simulink model "Praktikum06"  (R2023b)
settings: Solver=VariableStepAuto  StartTime=0.0  StopTime=0.01  RelTol=1e-3
model workspace (MAT data in the model file):
  CodeRate = 0.75
  M = 16
  PunctureVector = [1; 1; 0; 1; 0; 1]
  TracebackDepth = 48
  Trelli.numInputSymbols = 2
  Trelli.numOutputSymbols = 4
  Trelli.numStates = 64
  Trelli.nextStates = [0  32; 0  32; 1  33; 1  33; 2  34; 2  34; 3  35; 3  35; 4  36; 4  36; 5  37; 5  37; 6  38; 6  38; 7  39; 7  39; 8  40; 8  40; 9  41; 9  41; 10  42; 10  42; 11  43; 11  43; 12  44; 12  44; 13  45; 13  45; 14  46; 14  46; 15  47; 15  47; 16  48; 16  48; 17  49; 17  49; 18  50; 18  50; 19  51; 19  51; 20  52; 20  52; 21  53; 21  53; 22  54; 22  54; 23  55; 23  55; 24  56; 24  56; 25  57; 25  57; 26  58; 26  58; 27  59; 27  59; 28  60; 28  60; 29  61; 29  61; 30  62; 30  62; 31  63; 31  63]
  Trelli.outputs = [0  3; 3  0; 1  2; 2  1; 0  3; 3  0; 1  2; 2  1; 3  0; 0  3; 2  1; 1  2; 3  0; 0  3; 2  1; 1  2; 3  0; 0  3; 2  1; 1  2; 3  0; 0  3; 2  1; 1  2; 0  3; 3  0; 1  2; 2  1; 0  3; 3  0; 1  2; 2  1; 2  1; 1  2; 3  0; 0  3; 2  1; 1  2; 3  0; 0  3; 1  2; 2  1; 0  3; 3  0; 1  2; 2  1; 0  3; 3  0; 1  2; 2  1; 0  3; 3  0; 1  2; 2  1; 0  3; 3  0; 2  1; 1  2; 3  0; 0  3; 2  1; 1  2; 3  0; 0  3]
  Ts = 5e-08
undefined symbols (not defined in the file): doppler, magnitude
libraries: dspxfrm3 x3, commchan3 x2, commrflib2 x2, commcnvcod2 x2, commdigbbndam3 x2, dspindex x2, dspsigops x2, commrandsrc3 x1, commsink2 x1, dspstat3 x1, dspmathops x1, dspquant2 x1
settings Model: Creator=suttarar@hu-berlin.de  LastModifiedBy=suttarar@hu-berlin.de

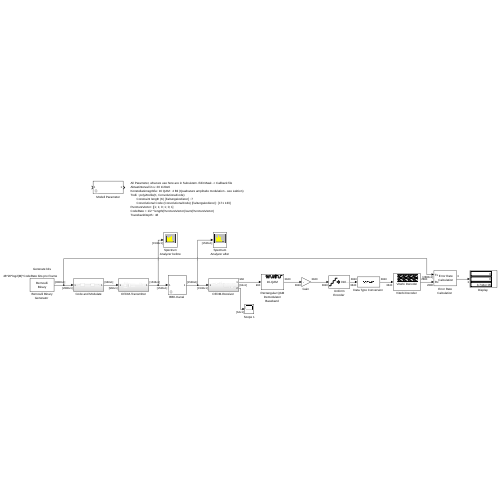
[thumbnail: Simulink's stored preview of the top-level diagram]
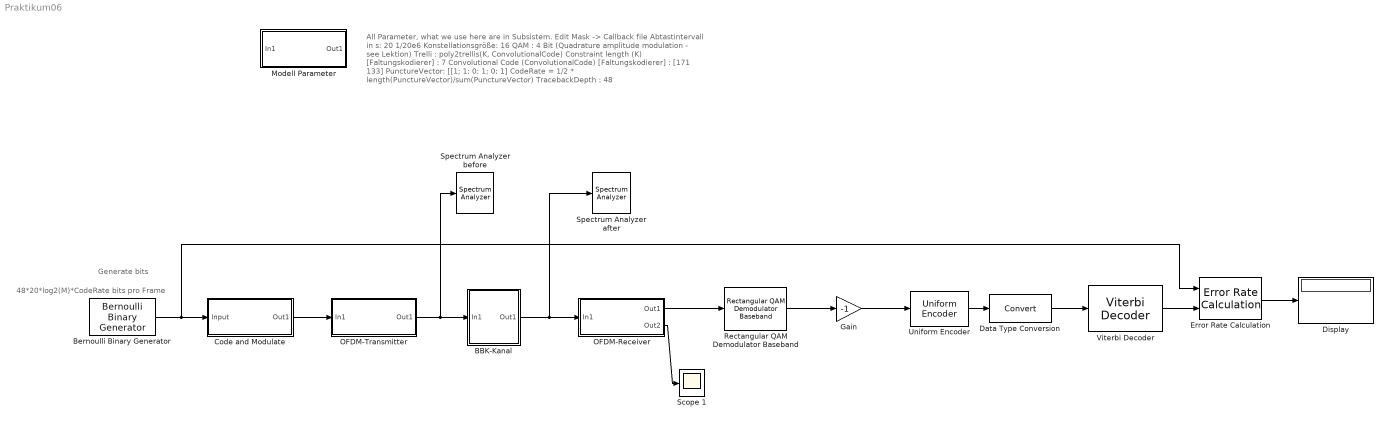
== system Praktikum06 ==
  note: All Parameter, what we use here are in Subsistem. Edit Mask -> Callback file
      | Abtastintervall in s: 20 1/20e6
      | Konstellationsgröße: 16 QAM : 4 Bit (Quadrature amplitude modulation - see Lektion)
      | Trelli : poly2trellis(K, ConvolutionalCode)
      | Constraint length (K) [Faltungskodierer] : 7
      | Convolutional Code (ConvolutionalCode) [Faltungskodierer] : [171 133]
      | PunctureVector: [[1; 1; 0; 1; 0; 1]
      | CodeRate = 1/2 * length(PunctureVector)/sum(PunctureVector)
      | TracebackDepth : 48
  note: 48*20*log2(M)*CodeRate bits pro Frame
  note: Generate bits
  "BBK-Kanal " : Subsystem  mask{MaxDoppler=0, PathDelays=0, PathGains=0, EnableMultipath=0, PathLoss=0, FrequencyOffset=0, PhaseOffset=0, SNR=15}
      mask prompts: MaxDoppler "Dopplerverschiebung"; PathDelays "Pfadverzoergerungen"; PathGains "Pfadverstaerkungen"; EnableMultipath "SwitchBlock"; PathLoss "Pfadverlust"; FrequencyOffset "Frequenzverschiebung"; PhaseOffset "Phasenverschiebung"; SNR "AWG-Rauschen"
  "Bernoulli Binary Generator " : commrandsrc3/Bernoulli Binary Generator  ProbabilityOfZero=0.5  SeedSource=Auto  Seed=0  SampleTime=Ts/(48*20*log2(M)*CodeRate)*64*24  SamplesPerFrame=48*20*log2(M)*CodeRate  OutputDataType=double  SimulateUsing=Interpreted execution
  Code and Modulate : Subsystem
  "Data Type Conversion " : DataTypeConversion  SaturateOnIntegerOverflow=off  RndMeth=Floor
  "Display " : Display
  "Error Rate Calculation " : commsink2/Error Rate Calculation  N=TracebackDepth  st_delay=48*20*log2(M)*CodeRate  cp_mode=Entire frame  subframe=[]  PMode=Port  WsName=ErrorVec  RsMode2=off  stop=off  numErr=100  maxBits=1e6
  "Gain " : Gain  Gain=-1
  Modell Parameter : Subsystem  mask{Ts=1/20e6, M=16, Trelli=poly2trellis(7, [171 133]), PunctureVector=[1; 1; 0; 1; 0; 1], CodeRate=0.75, TracebackDepth=48}
      mask prompts: Ts "Abtastintervall in s"; M "Konstellationsgröße"
  "OFDM-Receiver " : Subsystem
  OFDM-Transmitter : Subsystem
  "Rectangular QAM Demodulator Baseband " : commdigbbndam3/Rectangular QAM Demodulator Baseband  M=M  OutType=Bit  DecType=Approximate log-likelihood ratio  VarSource=Dialog  Variance=1  Dec=Gray  Mapping=[0:15]  PowType=Average Power  MinDist=2  AvgPow=1  PeakPow=1  Ph=0  outDtype1=Inherit via internal rule  outDtype2=Inherit via internal rule  derotateFactorWordLen=16  derotateFactorDataTypeStr=Inherit: Same word length as input  derotateFactorLastDataTypeStr=Inherit: Same word length as input  denormFactorWordLen=16  denormFactorDataTypeStr=Inherit: Same word length as input  denormFactorLastDataTypeStr=Inherit: Same word length as input  prodOutWordLen=32  prodOutOverflowMode=Wrap  prodOutRoundingMode=Floor  prodOutOvFlMode=off  prodOutOvFlModeLastStrValue=off  sumWordLen=32
  Scope 1 : Scope
  Spectrum Analyzer after : SpectrumAnalyzer  WindowPosition=[945.000000,268.000000,800.000000,500.000000,]  ScopeFrameLocation=window  YLimits=[-21.43598699,17.10318223]
  Spectrum Analyzer before : SpectrumAnalyzer  WindowPosition=[78.000000,269.000000,800.000000,500.000000,]  ScopeFrameLocation=window  YLimits=[-47.82803278,19.97346746]
  "Uniform Encoder " : dspquant2/Uniform Encoder  peak=1  bits=4  otype=Unsigned integer
  "Viterbi Decoder " : commcnvcod2/Viterbi Decoder  trellis=Trelli  isPunctured=on  punctureVector=PunctureVector  erasures=off  dectype=Soft decision  nsdecb=4  runSigValErrCheck=off  tbdepth=TracebackDepth  opmode=Continuous  reset=off  delayedResetAction=off  smWordLength=16  outDataType=double
  wires:
  Code and Modulate/1(Out1) -> OFDM-Transmitter/1(In1)
  "Rectangular QAM Demodulator Baseband "/1 -> "Gain "/1
  "Data Type Conversion "/1 -> "Viterbi Decoder "/1
  "OFDM-Receiver "/2(Out2) -> Scope 1/1
  "BBK-Kanal "/1(Out1) -> Spectrum Analyzer after/1, "OFDM-Receiver "/1(In1)
  OFDM-Transmitter/1(Out1) -> Spectrum Analyzer before/1, "BBK-Kanal "/1(In1)
  "Uniform Encoder "/1 -> "Data Type Conversion "/1
  "Viterbi Decoder "/1 -> "Error Rate Calculation "/2
  "OFDM-Receiver "/1(Out1) -> "Rectangular QAM Demodulator Baseband "/1
  "Error Rate Calculation "/1 -> "Display "/1
  "Gain "/1 -> "Uniform Encoder "/1
  "Bernoulli Binary Generator "/1 -> "Error Rate Calculation "/1, Code and Modulate/1(Input)

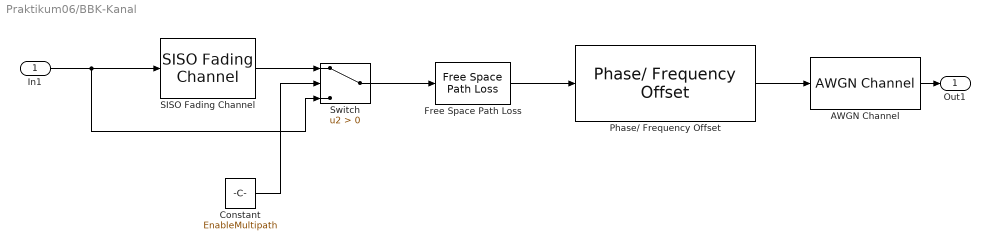
== system Praktikum06/BBK-Kanal  ==
  In1 : Inport
  AWGN Channel : commchan3/AWGN Channel  LegacyMode=off  NoiseMethod="Signal to noise ratio  (SNR)"  noiseMode="Signal to noise ratio  (SNR)"  EbNo=10  EsNo=10  SNR=SNR  BitsPerSymbol=1  SignalPower=1  SamplesPerSymbol=1  SymbolPeriod=1  VarianceSource=Parameter  Variance=1  RandomStream=Global stream  Seed=67  SimulateUsing=Code generation
  Constant : Constant  Value=EnableMultipath
  Free Space Path Loss : commrflib2/Free Space Path Loss  mode=Decibels  dB=PathLoss  d=0.100  fc=1920
  Phase/ Frequency Offset : commrflib2/Phase// Frequency Offset  phaseOffset=PhaseOffset  freqPort=off  freqOffset=FrequencyOffset
      settings: LibrarySourceBlock=|
      | commrfcorlib/Phase//
      | Frequency
      | Offset
  SISO Fading Channel : commchan3/SISO Fading Channel  InheritSampleRate=on  SampleRate=1  PathDelays=PathDelays  AveragePathGains=PathGains  NormalizePathGains=on  FadingDistribution=Rayleigh  KFactor=3  DirectPathDopplerShift=0  DirectPathInitialPhase=0  MaximumDopplerShift=MaxDoppler  DopplerSpectrum=doppler('Jakes')  RandomStream=mt19937ar with seed  Seed=73  PathGainsOutputPort=off  ChannelFilterDelayOutputPort=off  SimulateUsing=Interpreted execution  Visualization=Off  PathsForDopplerDisplay=1  SamplesToDisplay=25%
  Switch : Switch  Criteria=u2 > Threshold  SaturateOnIntegerOverflow=off  InputSameDT=off
  Out1 : Outport
  wires:
  Phase/ Frequency Offset/1 -> AWGN Channel/1
  Free Space Path Loss/1 -> Phase/ Frequency Offset/1
  AWGN Channel/1 -> Out1/1
  Switch/1 -> Free Space Path Loss/1
  SISO Fading Channel/1 -> Switch/1
  In1/1 -> Switch/3, SISO Fading Channel/1
  Constant/1 -> Switch/2

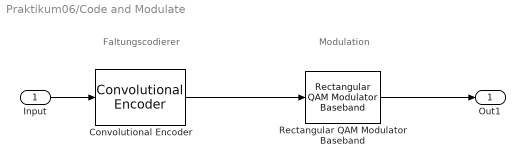
== system Praktikum06/Code and Modulate ==
  note: Modulation
  note: Faltungscodierer
  Input : Inport
  "Convolutional Encoder " : commcnvcod2/Convolutional Encoder  trellis=Trelli  opMode=Continuous  DelayedResetAction=off  hasIniStPort=off  hasFinStPort=off  usePuncVector=on  punctureVector=PunctureVector  reset=Unused parameter value
  "Rectangular QAM Modulator Baseband " : commdigbbndam3/Rectangular QAM Modulator Baseband  M=M  InType=Bit  Enc=Gray  Mapping=[0:15]  PowType=Average Power  MinDist=2  AvgPow=1  PeakPow=1  Ph=0  outDtype=double  outWordLen=16  outUDDataType=sfix(16)  outFracLenMode=Best precision  outFracLen=15  outDataTypeStr=double  outLastDataTypeStr=double
  Out1 : Outport
  wires:
  "Convolutional Encoder "/1 -> "Rectangular QAM Modulator Baseband "/1
  "Rectangular QAM Modulator Baseband "/1 -> Out1/1
  Input/1 -> "Convolutional Encoder "/1

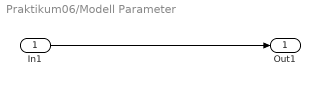
== system Praktikum06/Modell Parameter ==
  In1 : Inport
  Out1 : Outport
  wires:
  In1/1 -> Out1/1

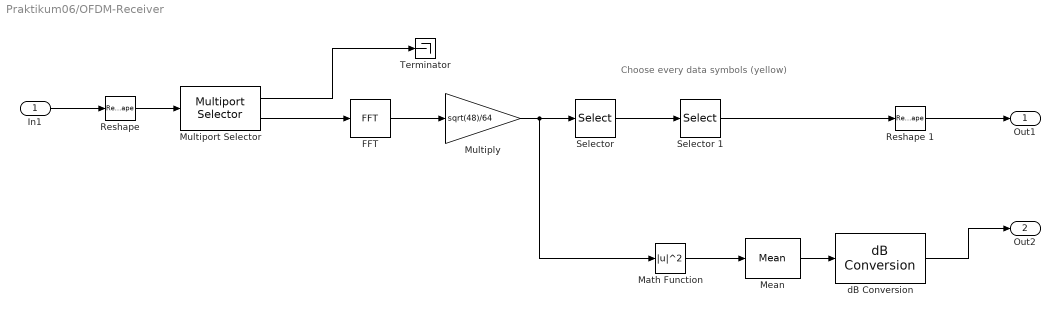
== system Praktikum06/OFDM-Receiver  ==
  note: Choose every data symbols (yellow)
  In1 : Inport
  "FFT " : dspxfrm3/FFT  FFTImplementation=Auto  CompMethod=Table lookup  TableOpt=NEW  TableOptActive=Speed  BitRevOrder=off  Normalize=off  InheritFFTLength=on  FFTLength=64  WrapInput=on  roundingMode=Floor  overflowMode=off  firstCoeffDataTypeStr=Inherit: Same word length as input  firstCoeffLastDataTypeStr=Inherit: Same word length as input  outputMin=[]  outputMax=[]
  "Math Function " : Math  Operator=magnitude^2
  "Mean " : dspstat3/Mean  run=off  InputProcessing=Columns as channels (frame based)  reset_popup=None  directionMode=Each row  dimension=1  roiEnable=off  roiType=Rectangles  roiPortion=Entire ROI  roiOutput=Individual statistics for each ROI  roiFlag=off  roundingMode=Floor  overflowMode=off  outputDataTypeStr=Inherit: Same as accumulator  outputMin=[]  outputMax=[]  outputLastDataTypeStr=Inherit: Same as accumulator
  "Multiply " : Gain  Gain=sqrt(48)/64
  "Multiport Selector " : dspindex/Multiport Selector  rowsOrCols=Columns  idxCellArray={[1:4], [5:24]}  idxErrMode=Clip Index
  "Reshape " : Reshape  OutputDimensionality=Customize  OutputDimensions=[64,24]
  Reshape 1 : Reshape  OutputDimensions=[64,24]
  "Selector " : Selector  NumberOfDimensions=2  InputPortWidth=3  IndexOptions=Index vector (dialog),Select all  Indices=[39:64 1:38],1  OutputSizes=1,1
  Selector 1 : Selector  NumberOfDimensions=2  InputPortWidth=3  IndexOptions=Index vector (dialog),Select all  Indices=[1:5 7:19 21:26 28:33 35:47 49:53],1  OutputSizes=1,1
  "Terminator " : Terminator
  "dB Conversion " : dspmathops/dB Conversion  dBtype=dB  intype=Power  R=1  fuzz=off
      settings: LibrarySourceBlock=commutil2/dB Conversion
  Out1 : Outport
  Out2 : Outport  Port=2
  wires:
  "Mean "/1 -> "dB Conversion "/1
  "Math Function "/1 -> "Mean "/1
  "FFT "/1 -> "Multiply "/1
  In1/1 -> "Reshape "/1
  "Selector "/1 -> Selector 1/1
  "Reshape "/1 -> "Multiport Selector "/1
  "Multiport Selector "/2 -> "FFT "/1
  "Multiport Selector "/1 -> "Terminator "/1
  "dB Conversion "/1 -> Out2/1
  Selector 1/1 -> Reshape 1/1
  Reshape 1/1 -> Out1/1
  "Multiply "/1 -> "Math Function "/1, "Selector "/1

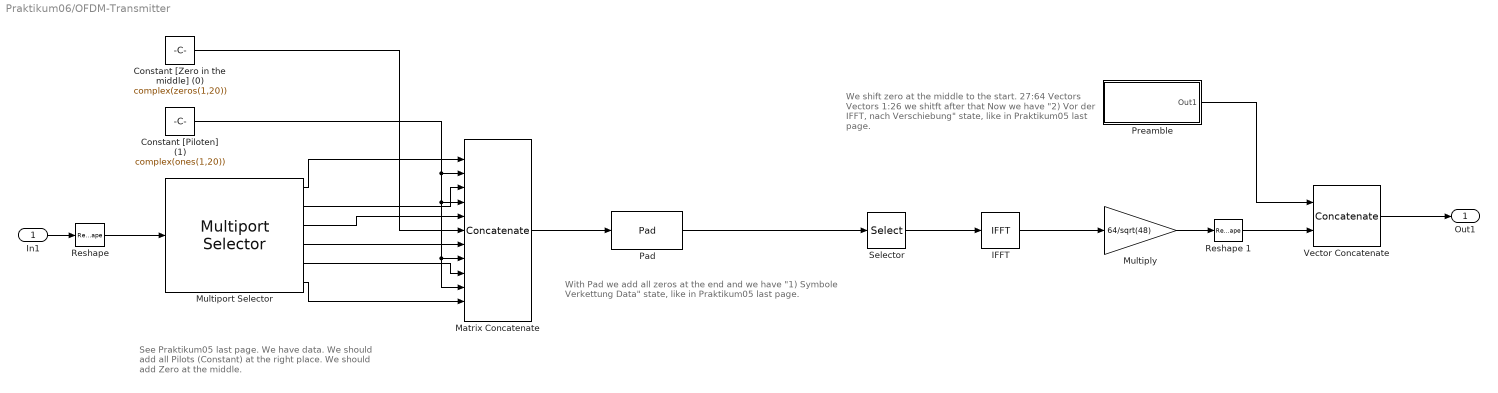
== system Praktikum06/OFDM-Transmitter ==
  note: With Pad we add all zeros at the end and we have
      | "1) Symbole Verkettung Data" state, like in Praktikum05 last page.
  note: See Praktikum05 last page. We have data.
      | We should add all Pilots (Constant) at the right place.
      | We should add Zero at the middle.
  note: We shift zero at the middle to the start.
      | 27:64 Vectors
      | Vectors 1:26 we shitft after that
      | Now we have "2) Vor der IFFT,
      | nach Verschiebung" state, like in Praktikum05 last page.
  In1 : Inport
  Constant [Piloten] (1) : Constant  Value=complex(ones(1,20))  VectorParams1D=off
  Constant [Zero in the middle] (0) : Constant  Value=complex(zeros(1,20))  VectorParams1D=off
  "IFFT " : dspxfrm3/IFFT  FFTImplementation=Auto  CompMethod=Table lookup  TableOpt=NEW  TableOptActive=Speed  BitRevOrder=off  cs_in=off  Normalize=on  InheritFFTLength=on  FFTLength=64  WrapInput=on  mode=Complex  outSamplingMode=Sample based  roundingMode=Floor  overflowMode=off  firstCoeffDataTypeStr=Inherit: Same word length as input  firstCoeffLastDataTypeStr=Inherit: Same word length as input  outputMin=[]  outputMax=[]
  "Matrix Concatenate " : Concatenate  NumInputs=11  Mode=Multidimensional array
  "Multiply " : Gain  Gain=64/sqrt(48)
  Multiport Selector : dspindex/Multiport Selector  rowsOrCols=Rows  idxCellArray={[1:5], [6:18], [19:24], [25:30], [31:43], [44:48]}  idxErrMode=Clip Index
      settings: LibrarySourceBlock=|
      | dsphdlsupportsigmgmt/Multiport
      | Selector
  "Pad " : dspsigops/Pad  padAlong=Columns  dimsToPad=1  valSrc=Specify via dialog  padVal=0  spec=Output size  padNumOutRowsSpecMethod=User-specified  numOutRows=64  padNumOutColsSpecMethod=User-specified  numOutCols=1  isVarDimsMode=off  padBeginning=0  padEnd=0  outSizeMode=User-specified  outSize=1  padSigAt=End  trunc_flag=None  roundingMode=Floor  overflowMode=off  truncOrWrapMode=Truncate  wrap_flag=None
  Preamble : Subsystem
  "Reshape " : Reshape  OutputDimensionality=Customize  OutputDimensions=[48,20]
  Reshape 1 : Reshape  OutputDimensionality=Column vector (2-D)  OutputDimensions=[64,24]
  "Selector " : Selector  NumberOfDimensions=2  InputPortWidth=3  IndexOptions=Index vector (dialog),Select all  Indices=[27:64 1:26],1  OutputSizes=1,1
  Vector Concatenate : Concatenate
  Out1 : Outport
  wires:
  In1/1 -> "Reshape "/1
  "Reshape "/1 -> Multiport Selector/1
  "Pad "/1 -> "Selector "/1
  "Matrix Concatenate "/1 -> "Pad "/1
  Multiport Selector/1 -> "Matrix Concatenate "/1
  Multiport Selector/2 -> "Matrix Concatenate "/3
  Multiport Selector/3 -> "Matrix Concatenate "/5
  Multiport Selector/4 -> "Matrix Concatenate "/7
  Multiport Selector/5 -> "Matrix Concatenate "/9
  Multiport Selector/6 -> "Matrix Concatenate "/11
  Constant [Piloten] (1)/1 -> "Matrix Concatenate "/10, "Matrix Concatenate "/8, "Matrix Concatenate "/4, "Matrix Concatenate "/2
  Constant [Zero in the middle] (0)/1 -> "Matrix Concatenate "/6
  "Selector "/1 -> "IFFT "/1
  "IFFT "/1 -> "Multiply "/1
  "Multiply "/1 -> Reshape 1/1
  Reshape 1/1 -> Vector Concatenate/2
  Vector Concatenate/1 -> Out1/1
  Preamble/1(Out1) -> Vector Concatenate/1

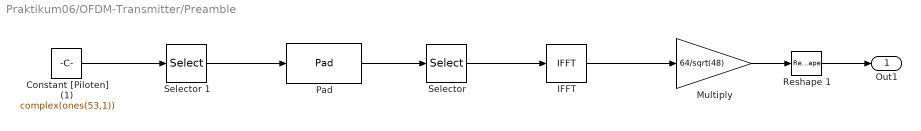
== system Praktikum06/OFDM-Transmitter/Preamble ==
  Constant [Piloten] (1) : Constant  Value=complex(ones(53,1))  VectorParams1D=off
  "IFFT " : dspxfrm3/IFFT  FFTImplementation=Auto  CompMethod=Table lookup  TableOpt=NEW  TableOptActive=Speed  BitRevOrder=off  cs_in=off  Normalize=on  InheritFFTLength=on  FFTLength=64  WrapInput=on  mode=Complex  outSamplingMode=Sample based  roundingMode=Floor  overflowMode=off  firstCoeffDataTypeStr=Inherit: Same word length as input  firstCoeffLastDataTypeStr=Inherit: Same word length as input  outputMin=[]  outputMax=[]
  "Multiply " : Gain  Gain=64/sqrt(48)
  "Pad " : dspsigops/Pad  padAlong=Columns  dimsToPad=1  valSrc=Specify via dialog  padVal=0  spec=Output size  padNumOutRowsSpecMethod=User-specified  numOutRows=64  padNumOutColsSpecMethod=User-specified  numOutCols=1  isVarDimsMode=off  padBeginning=0  padEnd=0  outSizeMode=User-specified  outSize=1  padSigAt=End  trunc_flag=None  roundingMode=Floor  overflowMode=off  truncOrWrapMode=Truncate  wrap_flag=None
  Reshape 1 : Reshape  OutputDimensionality=Column vector (2-D)  OutputDimensions=[64,24]
  "Selector " : Selector  NumberOfDimensions=2  InputPortWidth=3  IndexOptions=Index vector (dialog),Select all  Indices=[27:64 1:26],1  OutputSizes=1,1
  Selector 1 : Selector  NumberOfDimensions=2  InputPortWidth=3  IndexOptions=Select all,Index vector (dialog)  Indices=[27:64 1:26],[1 1 1 1]  OutputSizes=1,1
  Out1 : Outport
  wires:
  "Pad "/1 -> "Selector "/1
  "Selector "/1 -> "IFFT "/1
  "Multiply "/1 -> Reshape 1/1
  "IFFT "/1 -> "Multiply "/1
  Reshape 1/1 -> Out1/1
  Constant [Piloten] (1)/1 -> Selector 1/1
  Selector 1/1 -> "Pad "/1
